simulink model "task2"  (R2021a)
settings: Solver=FixedStepDiscrete  StartTime=0.0  StopTime=10.0  RelTol=1e-3  EnableMultiTasking=on
settings Model: Creator=Karim  LastModifiedBy=Karim
settings DataIOCC: ReturnWorkspaceOutputs=off
settings OptimizationCC: DefaultParameterBehavior=Inlined  InlineInvariantSignals=on  EnableMemcpy=off  LifeSpan=1  EfficientTunableParamExpr=on
settings DebuggingCC: UnderspecifiedInitializationDetection=Classic  MergeDetectMultiDrivingBlocksExec=none  SFMachineParentedDataDiag=warning  ArithmeticOperatorsInVariantConditions=warning
settings ModelReferenceCC: PropagateSignalLabelsOutOfModel=off
settings SFSimCC: MATLABDynamicMemAlloc=off  CustomCodeUndefinedFunction=UseInterfaceOnly
settings RTWCC: SystemTargetFile=ert.tlc  GenCodeOnly=on  TemplateMakefile=ert_default_tmf  GenerateReport=on  IncludeHyperlinkInReport=on  LaunchReport=on  GenerateTraceInfo=on  GenerateTraceReport=on  GenerateTraceReportSl=on  GenerateTraceReportSf=on  GenerateTraceReportEml=on
settings CodeAppCC: ForceParamTrailComments=on  IgnoreCustomStorageClasses=off  OperatorAnnotations=on  SimulinkDataObjDesc=on  SFDataObjDesc=on  MATLABFcnDesc=on  InsertBlockDesc=on  StateflowObjectComments=on  MATLABSourceComments=on
settings ERTTargetCC: MultiwordLength=2048  GenerateSampleERTMain=on  InlinedParameterPlacement=NonHierarchical  ERTCustomFileTemplate=example_file_process.tlc

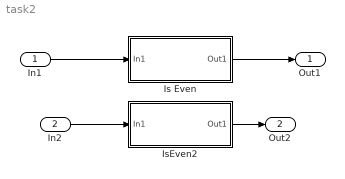
== system task2 ==
  In1 : Inport
  In2 : Inport  Port=2
  Is Even : Subsystem
  IsEven2 : Subsystem
  Out1 : Outport
  Out2 : Outport  Port=2
  wires:
  In1/1 -> Is Even/1(In1)
  Is Even/1(Out1) -> Out1/1
  IsEven2/1(Out1) -> Out2/1
  In2/1 -> IsEven2/1(In1)

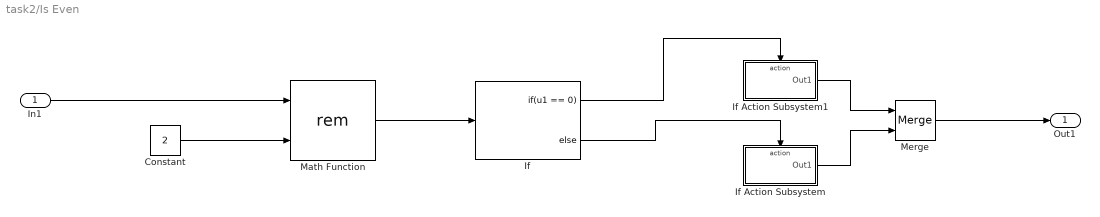
== system task2/Is Even ==
  In1 : Inport
  Constant : Constant  Value=2
  If : If  IfExpression=u1 == 0
  If Action Subsystem : Subsystem  TreatAsAtomicUnit=on
  If Action Subsystem1 : Subsystem  TreatAsAtomicUnit=on
  Math Function : Math  Operator=rem  SaturateOnIntegerOverflow=on
  Merge : Merge
  Out1 : Outport
  wires:
  If/2 -> If Action Subsystem/Action
  If/1 -> If Action Subsystem1/Action
  Math Function/1 -> If/1
  Constant/1 -> Math Function/2
  If Action Subsystem/1(Out1) -> Merge/2
  If Action Subsystem1/1(Out1) -> Merge/1
  In1/1 -> Math Function/1
  Merge/1 -> Out1/1

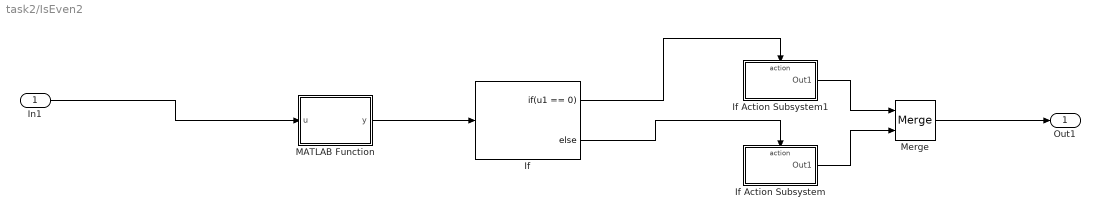
== system task2/IsEven2 ==
  In1 : Inport
  If : If  IfExpression=u1 == 0
  If Action Subsystem : Subsystem  TreatAsAtomicUnit=on
  If Action Subsystem1 : Subsystem  TreatAsAtomicUnit=on
  MATLAB Function : MATLAB Function  TreatAsAtomicUnit=on
  Merge : Merge
  Out1 : Outport
  wires:
  If Action Subsystem1/1(Out1) -> Merge/1
  MATLAB Function/1(y) -> If/1
  If/2 -> If Action Subsystem/Action
  In1/1 -> MATLAB Function/1(u)
  If/1 -> If Action Subsystem1/Action
  Merge/1 -> Out1/1
  If Action Subsystem/1(Out1) -> Merge/2

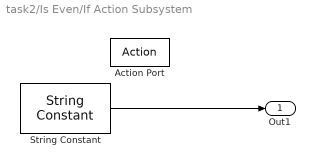
== system task2/Is Even/If Action Subsystem ==
  Action Port : ActionPort  ActionPortLabel=else
  String Constant : StringConstant  String="\"odd\""
  Out1 : Outport
  wires:
  String Constant/1 -> Out1/1

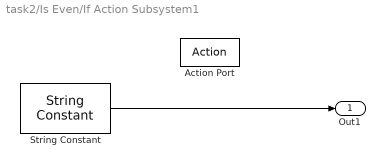
== system task2/Is Even/If Action Subsystem1 ==
  Action Port : ActionPort  ActionPortLabel=if(u1 == 0)
  String Constant : StringConstant  String="\"Even\""
  Out1 : Outport
  wires:
  String Constant/1 -> Out1/1

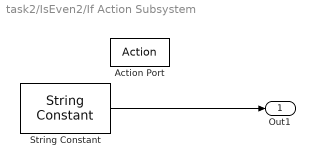
== system task2/IsEven2/If Action Subsystem ==
  Action Port : ActionPort  ActionPortLabel=else
  String Constant : StringConstant  String="\"odd\""
  Out1 : Outport
  wires:
  String Constant/1 -> Out1/1

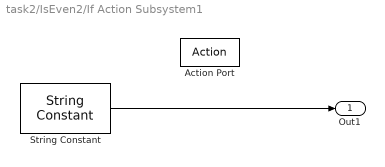
== system task2/IsEven2/If Action Subsystem1 ==
  Action Port : ActionPort  ActionPortLabel=if(u1 == 0)
  String Constant : StringConstant  String="\"Even\""
  Out1 : Outport
  wires:
  String Constant/1 -> Out1/1

== matlab function task2/IsEven2/MATLAB Function ==
  data: u input; y output
function y = fcn(u)

y = u%2;
end
